simulink model "prelab_9"  (R2014a)
settings: Solver=FixedStepDiscrete  StartTime=0.0  StopTime=1000000  FixedStep=1  RelTol=1e-3
libraries: hdlsllib x5, simulink x2
settings Model: Creator=liu.xind  LastModifiedBy=fan.x
settings OptimizationCC: BlockReduction=off  ConditionallyExecuteInputs=off  InlineParams=on
settings DebuggingCC: AlgebraicLoopMsg=error  MergeDetectMultiDrivingBlocksExec=error
settings HardwareCC: ProdHWDeviceType=ASIC/FPGA->ASIC/FPGA  ProdEqTarget=off

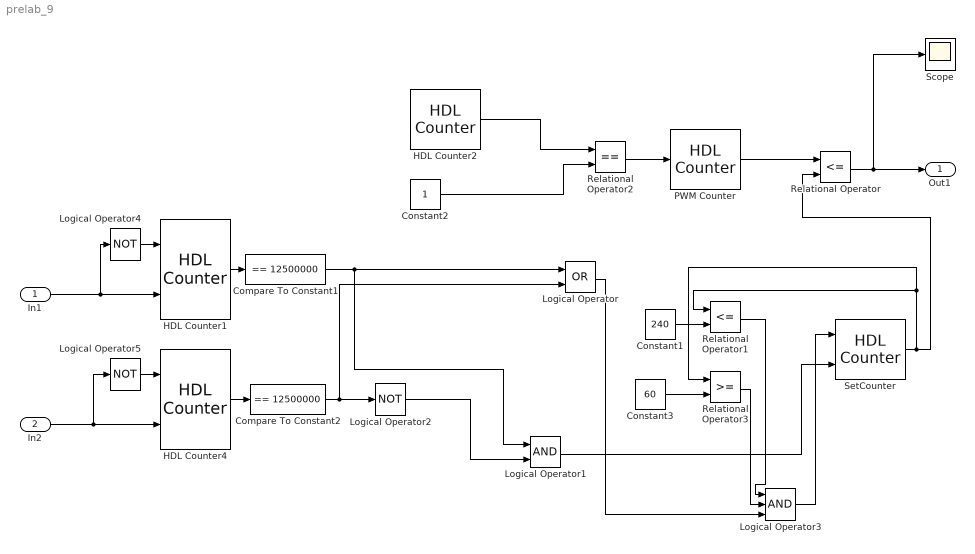
== system prelab_9 ==
  In1 : Inport  OutDataTypeStr=boolean
  In2 : Inport  Port=2  OutDataTypeStr=boolean
  Compare To Constant1 : simulink/Logic and Bit Operations/Compare To Constant  relop===  const=12500000  OutDataTypeStr=boolean
  Compare To Constant2 : simulink/Logic and Bit Operations/Compare To Constant  relop===  const=12500000  OutDataTypeStr=boolean
  Constant1 : Constant  Value=240  OutDataTypeStr=uint8
  Constant2 : Constant  OutDataTypeStr=uint8
  Constant3 : Constant  Value=60  OutDataTypeStr=uint8
  HDL Counter1 : hdlsllib/HDL Operations/HDL Counter  CountType=Count limited  CountInit=0  CountStep=1  CountMax=50000000  CountFromType=Initial value  CountFrom=0  CountResetPort=on  CountLoadPort=off  CountEnbPort=on  CountDirPort=off  CountDataType=Unsigned  CountWordLen=32  CountFracLen=0  CountSampTime=1
  HDL Counter2 : hdlsllib/HDL Operations/HDL Counter  CountType=Count limited  CountInit=0  CountStep=1  CountMax=500  CountFromType=Initial value  CountFrom=0  CountResetPort=off  CountLoadPort=off  CountEnbPort=off  CountDirPort=off  CountDataType=Unsigned  CountWordLen=32  CountFracLen=0  CountSampTime=1
  HDL Counter4 : hdlsllib/HDL Operations/HDL Counter  CountType=Count limited  CountInit=0  CountStep=1  CountMax=50000000  CountFromType=Initial value  CountFrom=0  CountResetPort=on  CountLoadPort=off  CountEnbPort=on  CountDirPort=off  CountDataType=Unsigned  CountWordLen=32  CountFracLen=0  CountSampTime=1
  Logical Operator : Logic  Operator=OR  AllPortsSameDT=off  OutDataTypeStr=boolean
  Logical Operator1 : Logic  AllPortsSameDT=off  OutDataTypeStr=boolean
  Logical Operator2 : Logic  Operator=NOT  AllPortsSameDT=off  OutDataTypeStr=boolean
  Logical Operator3 : Logic  Inputs=3  AllPortsSameDT=off  OutDataTypeStr=boolean
  Logical Operator4 : Logic  Operator=NOT  AllPortsSameDT=off  OutDataTypeStr=boolean
  Logical Operator5 : Logic  Operator=NOT  AllPortsSameDT=off  OutDataTypeStr=boolean
  PWM Counter : hdlsllib/HDL Operations/HDL Counter  CountType=Count limited  CountInit=0  CountStep=1  CountMax=2000  CountFromType=Initial value  CountFrom=0  CountResetPort=off  CountLoadPort=off  CountEnbPort=on  CountDirPort=off  CountDataType=Unsigned  CountWordLen=16  CountFracLen=0  CountSampTime=1
  Relational Operator : RelationalOperator  Operator=<=  OutDataTypeStr=boolean
  Relational Operator1 : RelationalOperator  Operator=<=  OutDataTypeStr=boolean
  Relational Operator2 : RelationalOperator  Operator===  OutDataTypeStr=boolean
  Relational Operator3 : RelationalOperator  OutDataTypeStr=boolean
  Scope : Scope
  SetCounter : hdlsllib/HDL Operations/HDL Counter  CountType=Count limited  CountInit=150  CountStep=12  CountMax=240  CountFromType=Initial value  CountFrom=150  CountResetPort=off  CountLoadPort=off  CountEnbPort=on  CountDirPort=on  CountDataType=Unsigned  CountWordLen=8  CountFracLen=0  CountSampTime=1
  Out1 : Outport  OutDataTypeStr=boolean
  wires:
  PWM Counter/1 -> Relational Operator/1
  Relational Operator/1 -> Scope/1, Out1/1
  HDL Counter2/1 -> Relational Operator2/1
  Constant2/1 -> Relational Operator2/2
  Relational Operator2/1 -> PWM Counter/1
  Logical Operator1/1 -> SetCounter/2
  Logical Operator2/1 -> Logical Operator1/2
  Constant1/1 -> Relational Operator1/2
  SetCounter/1 -> Relational Operator1/1, Relational Operator3/1, Relational Operator/2
  Constant3/1 -> Relational Operator3/2
  Relational Operator1/1 -> Logical Operator3/1
  Relational Operator3/1 -> Logical Operator3/2
  Logical Operator3/1 -> SetCounter/1
  Compare To Constant1/1 -> Logical Operator1/1, Logical Operator/1
  Compare To Constant2/1 -> Logical Operator/2, Logical Operator2/1
  In1/1 -> Logical Operator4/1, HDL Counter1/2
  Logical Operator4/1 -> HDL Counter1/1
  HDL Counter1/1 -> Compare To Constant1/1
  In2/1 -> Logical Operator5/1, HDL Counter4/2
  Logical Operator5/1 -> HDL Counter4/1
  HDL Counter4/1 -> Compare To Constant2/1
  Logical Operator/1 -> Logical Operator3/3
